simulink model "Mcity"  (R2019a)
settings: Solver=VariableStepAuto  StartTime=0.0  StopTime=100  RelTol=1e-3
undefined symbols (not defined in the file or in its folder): m, n
settings Model: Creator=nebneBgnahZ  LastModifiedBy=nebneBgnahZ
settings DataIOCC: ReturnWorkspaceOutputs=off
settings DebuggingCC: ArithmeticOperatorsInVariantConditions=warning
settings SFSimCC: SimUseLocalCustomCode=off
settings RTWCC: RTWUseLocalCustomCode=off
settings CodeAppCC: StateflowObjectComments=on

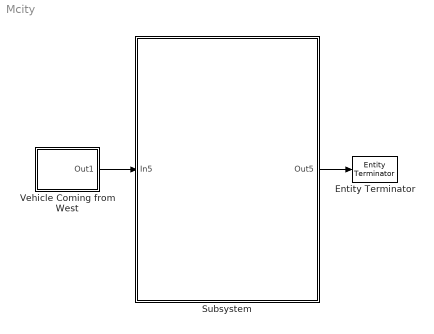
== system Mcity ==
  Entity Terminator : EntityTerminator  InputPortMessageModes=m
      mask Display: image('figs/CAV2.png');
  Subsystem : Subsystem
      mask Display: image('figs/Mcity Map - High Res.jpg');
  Vehicle Coming from West : Subsystem  mask(Connected Automated Vehicles (CAVs)){modelpopup=Basic model, umin=[], umax=[], vmin=[], vmax=[], length=0, cf=0, cr=0, lf=0, lr=0}
      mask prompts: modelpopup "Vehicle Model Selection"; umin "Maximum Deceleration"; umax "Maximum Acceleration"; vmin "Minimum Speed"; vmax "Maximum Speed"; cf "Front Tire Cornering Stiffness"; cr "Rear Tire Cornering Stiffness"; lf "Distance from CoG to Front Axels"; lr "Distance from CoG to Rear Axels"
      mask help: Vehicles, assumed to be CAVs, should possess the ability to communicate with the controller, the coordinator, and other vehicles in the network. CAVs can differ in driver models, for instance, motion dynamics, control mechanism, and fuel consumption dynamics.
      mask TypeOptions modelpopup: Basic model | Kinematic model | Dynamic model | User-defined
      mask Callback modelpopup:
      | % Get the mask parameter values. This is a cell
      | %   array of character vectors.
      | maskStr = get_param(gcb,'modelpopup');
      | 
      | % The pop-up menu is the first mask parameter.
      | %   Check the value selected in the pop-up
      | if strcmp(maskStr(1),'U')
      | 
      | 
      |     % Set the visibility of both parameters on when
      |     %   User-defined is selected in the pop-up.
      | 
      |     set_param(gcb,'MaskVisibilities',{'on';'on';'on';'on';'on';'on';'on';'on';'on';'on';}),
      | 
      | elseif strcmp(maskStr(1),'B')
      | 
      |     % Turn off the visibility of the Value field
      |     %   when User-defined is not selected.
      | 
      |     set_param(gcb,'MaskVisibilities',{'on';'on';'on';'on';'on';'off';'off';'off';'off';'off';}),
      | 
      |     % Set the character vector in the Values field equal to the
      |     % character vector selected in the Gain pop-up menu.
      | 
      |     %maskStr{2}=maskStr{1};
      | 
      | 
      | elseif strcmp(maskStr(1),'K')
      | 
      |     set_param(gcb,'MaskVisibilities',{'on';'on';'on';'on';'on';'on';'off';'off';'off';'off';}),
      | 
      | else
      | 
      |     set_param(gcb,'MaskVisibilities',{'on';'on';'on';'on';'on';'off';'on';'on';'on';'on';}),
      | 
      | end
      mask Display: image('figs/CAV.png');
  wires:
  Subsystem/1(Out5) -> Entity Terminator/1
  Vehicle Coming from West/1(Out1) -> Subsystem/1(In5)

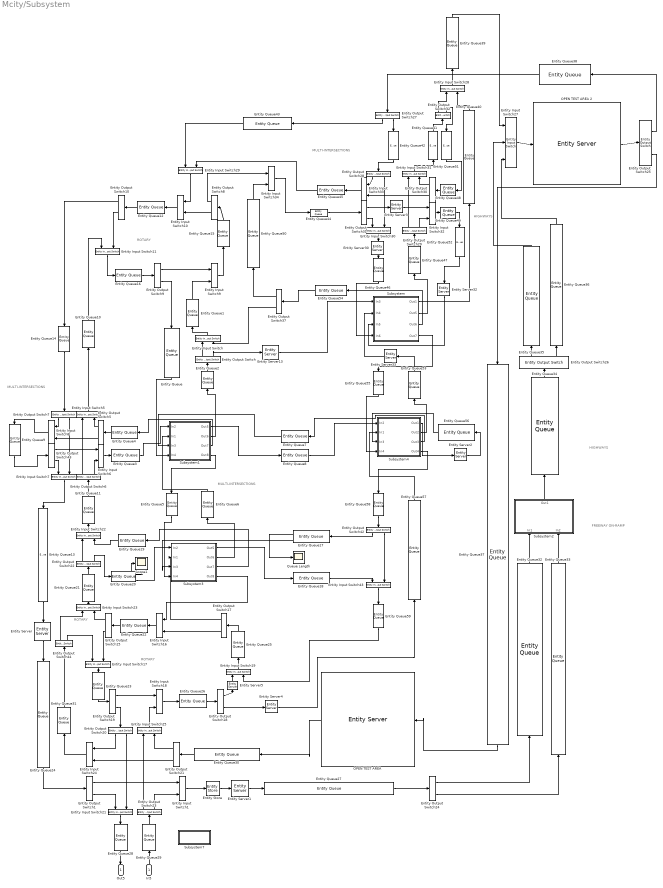
== system Mcity/Subsystem ==
  note: FREEWAY
      | ON-RAMP
  note: HIGHWAYS
  note: MULTI-INTERSECTIONS
  note: ROTARY
  note: ROTARY
  note: ROTARY
  note: MULTI-INTERSECTIONS
  note: MULTI-INTERSECTIONS
  note: HIGHWAYS
  In5 : Inport
  Entity Input Switch{,1,5..11,16..19,21..25,28..34,43} (26 alike) : EntityInputSwitch  InputPortMessageModes=m,m  OutputPortMessageModes=m
  Entity Input Switch27 : EntityInputSwitch  InputPortMessageModes=m,m,m  OutputPortMessageModes=m  NumberInputPorts=3
      settings: InputPortMap=u1,u2,u3
  Entity Output Switch{,1,5..10,15,18,20..22,24..32,37,42..44} (26 alike) : EntityOutputSwitch  InputPortMessageModes=m  OutputPortMessageModes=m,m  SwitchingCriterion=Round robin  SwitchAttributeName=Attribute1
  Entity Output Switch17 : EntityOutputSwitch  InputPortMessageModes=m  OutputPortMessageModes=m,m  SwitchAttributeName=Attribute1
  Entity Output Switch19 : EntityOutputSwitch  InputPortMessageModes=m  OutputPortMessageModes=m,m  SwitchAttributeName=Attribute1
  Entity Output Switch23 : EntityOutputSwitch  InputPortMessageModes=m  OutputPortMessageModes=m,m  SwitchingCriterion=Round robin  SwitchAttributeName=Lane
  Entity Queue{,1..16,19,21..26,28,30..31,35..59} (52 alike) : EntityQueue  InputPortMessageModes=m  OutputPortMessageModes=m
      settings: OutputPortMap=o5
  Entity Queue17 : EntityQueue  InputPortMessageModes=m  OutputPortMessageModes=n,m  Capacity=15  NumberEntitiesInBlock=on
      settings: OutputPortMap=o1,o5
  Entity Queue18 : EntityQueue  InputPortMessageModes=m  OutputPortMessageModes=m  Capacity=15
      settings: OutputPortMap=o5
  Entity Queue20 : EntityQueue  InputPortMessageModes=m  OutputPortMessageModes=n,m  AverageQueueLength=on
      settings: OutputPortMap=o3,o5
  Entity Queue{27,29,32..34} (5 alike) : EntityQueue  InputPortMessageModes=m  OutputPortMessageModes=m  Capacity=Inf
      settings: OutputPortMap=o5
  Entity Server{,3,5,13,30,32..33} (7 alike) : EntityServer  InputPortMessageModes=m  OutputPortMessageModes=m  Capacity=Inf  ServiceTimeValue=2.5
  Entity Server1 : EntityServer  InputPortMessageModes=m  OutputPortMessageModes=m  Capacity=1  ServiceTimeValue=2
  Entity Server2 : EntityServer  InputPortMessageModes=m  OutputPortMessageModes=m  Capacity=Inf  ServiceTimeValue=5
  Entity Server4 : EntityServer  InputPortMessageModes=m  OutputPortMessageModes=m  Capacity=Inf  ServiceTimeValue=5
  Entity Store : EntityStore  InputPortMessageModes=m  OutputPortMessageModes=m  Capacity=100
      settings: OutputPortMap=o4
  OPEN TEST AREA : EntityServer  InputPortMessageModes=m  OutputPortMessageModes=m  Capacity=200
  "OPEN TEST AREA 2 " : EntityServer  InputPortMessageModes=m  OutputPortMessageModes=m  Capacity=200
  Queue Length : Scope
  Scope1 : Scope
  Subsystem : Subsystem
      mask Display:
      | %image('figs/tlc.png');
      | 
      | fprintf('Signalized\n\n');
      | fprintf('\n\nIntersection 1');
  Subsystem1 : Subsystem
      mask Display:
      | %image('figs/unsignalized.png');
      | fprintf('Unsignalized\n\n');
      | fprintf('\n\nIntersection 1');
  Subsystem2 : Subsystem
      mask Display:
      | %image('figs/merge.png');
      | %image('figs/unsignalized.png');
      | fprintf('Freeway\n\n');
      | fprintf('\n\n On-Ramp');
  Subsystem3 : Subsystem
      mask Display:
      | %image('figs/tlc.png');
      | fprintf('Signalized\n\n');
      | fprintf('\n\nIntersection 2');
  Subsystem4 : Subsystem
      mask Display:
      | %image('figs/unsignalized.png');
      | fprintf('Unsignalized\n\n');
      | fprintf('\n\nIntersection 2');
  Subsystem7 : Subsystem
      settings: OpenFcn=init_func
      mask Display: disp('init');
  Out5 : Outport
  wires:
  Subsystem1/4(Out8) -> Entity Queue5/1
  Entity Input Switch10/1 -> Entity Queue12/1
  Entity Output Switch8/2 -> Entity Input Switch10/2
  Entity Output Switch24/1 -> Entity Queue32/1
  Entity Output Switch24/2 -> Entity Queue33/1
  Entity Queue34/1 -> Entity Output Switch26/1
  Entity Output Switch26/1 -> Entity Queue35/1
  Entity Output Switch26/2 -> Entity Queue36/1
  Entity Input Switch27/1 -> "OPEN TEST AREA 2 "/1
  "OPEN TEST AREA 2 "/1 -> Entity Output Switch25/1
  Entity Queue37/1 -> OPEN TEST AREA/1
  Entity Output Switch25/1 -> Entity Queue38/1
  Entity Queue36/1 -> Entity Input Switch27/3
  Entity Queue35/1 -> Entity Input Switch27/2
  Entity Queue39/1 -> Entity Input Switch27/1
  Entity Input Switch28/1 -> Entity Queue39/1
  Entity Queue40/1 -> Entity Input Switch28/2
  Entity Queue41/1 -> Entity Output Switch32/1
  Entity Queue38/1 -> Entity Output Switch27/1
  Entity Output Switch27/1 -> Entity Queue43/1
  Entity Output Switch27/2 -> Entity Queue42/1
  Entity Input Switch29/1 -> Entity Input Switch10/1
  Entity Queue43/1 -> Entity Input Switch29/1
  Entity Output Switch31/2 -> Entity Input Switch30/1
  Entity Output Switch31/1 -> Entity Server3/1
  Entity Input Switch33/1 -> Entity Queue45/1
  Entity Output Switch28/1 -> Entity Input Switch33/1
  Entity Output Switch30/1 -> Entity Input Switch31/2
  Entity Output Switch30/2 -> Entity Input Switch33/2
  Entity Output Switch29/1 -> Entity Input Switch31/1
  Entity Input Switch32/1 -> Entity Queue49/1
  Entity Queue48/1 -> Entity Output Switch30/1
  Entity Output Switch29/2 -> Entity Input Switch32/2
  Entity Queue45/1 -> Entity Input Switch29/2
  Entity Queue47/1 -> Entity Output Switch29/1
  Entity Queue42/1 -> Entity Output Switch28/1
  Entity Input Switch31/1 -> Entity Queue41/1
  Entity Queue50/1 -> Entity Input Switch34/2
  Entity Input Switch34/1 -> Entity Queue44/1
  Entity Output Switch32/1 -> Entity Input Switch28/1
  Entity Output Switch32/2 -> Entity Queue51/1
  Entity Queue51/1 -> Entity Queue48/1
  Entity Queue49/1 -> Entity Queue52/1
  Entity Queue54/1 -> Entity Output Switch37/1
  Entity Output Switch37/1 -> Entity Queue50/1
  Subsystem4/2(Out2) -> Entity Queue53/1
  Subsystem4/1(Out1) -> Entity Server2/1
  Subsystem4/4(Out4) -> Entity Queue58/1
  Entity Queue58/1 -> Entity Output Switch42/1
  Entity Input Switch43/1 -> Entity Queue59/1
  Entity Output Switch8/1 -> Entity Input Switch34/1
  Entity Output Switch10/2 -> Entity Input Switch11/2
  Entity Input Switch11/1 -> Entity Queue16/1
  Entity Queue16/1 -> Entity Output Switch9/1
  Entity Queue12/1 -> Entity Output Switch10/1
  Entity Queue15/1 -> Entity Output Switch8/1
  Entity Input Switch9/1 -> Entity Queue15/1
  Entity Input Switch16/1 -> Entity Queue22/1
  Entity Queue22/1 -> Entity Output Switch15/1
  Entity Input Switch17/1 -> Entity Queue23/1
  Entity Output Switch17/2 -> Entity Input Switch16/2
  Entity Queue26/1 -> Entity Output Switch18/1
  Entity Queue23/1 -> Entity Output Switch19/1
  Entity Input Switch19/1 -> Entity Queue25/1
  Entity Queue25/1 -> Entity Output Switch17/1
  Entity Queue30/1 -> Entity Output Switch21/1
  Entity Input Switch22/1 -> Entity Queue11/1
  Entity Output Switch22/1 -> Entity Input Switch22/1
  Entity Queue21/1 -> Entity Output Switch22/1
  Entity Input Switch23/1 -> Entity Queue21/1
  Entity Output Switch15/1 -> Entity Input Switch23/2
  Entity Queue31/1 -> Entity Output Switch44/1
  Entity Queue29/1 -> Entity Output Switch23/1
  Entity Input Switch21/1 -> Entity Queue28/1
  Entity Queue28/1 -> Out5/1
  In5/1 -> Entity Queue29/1
  Entity Output Switch5/2 -> Entity Input Switch8/2
  Entity Input Switch7/1 -> Entity Queue13/1
  Entity Output Switch7/2 -> Entity Input Switch7/2
  Entity Output Switch6/1 -> Entity Input Switch5/1
  Entity Output Switch9/1 -> Entity Input Switch9/1
  Entity Input Switch/1 -> Entity Queue1/1
  Subsystem1/2(Out6) -> Entity Queue2/1
  Entity Output Switch37/2 -> Entity Input Switch/2
  Entity Output Switch/2 -> Entity Server13/1
  Subsystem1/3(Out7) -> Entity Queue4/1
  Entity Queue2/1 -> Entity Output Switch/1
  Entity Output Switch9/2 -> Entity Queue/1
  Entity Queue1/1 -> Entity Input Switch9/2
  Entity Queue7/1 -> Subsystem1/3(In3)
  Entity Output Switch/1 -> Entity Input Switch/1
  Entity Queue4/1 -> Entity Output Switch5/1
  Entity Input Switch5/1 -> Entity Queue10/1
  Entity Output Switch5/1 -> Entity Input Switch5/2
  Entity Input Switch6/1 -> Entity Queue3/1
  Entity Output Switch6/2 -> Entity Input Switch6/2
  Entity Queue11/1 -> Entity Output Switch6/1
  Entity Queue9/1 -> Entity Output Switch43/1
  Entity Output Switch7/1 -> Entity Input Switch8/1
  Entity Queue14/1 -> Entity Output Switch7/1
  Entity Output Switch43/1 -> Entity Input Switch6/1
  Entity Output Switch43/2 -> Entity Input Switch7/1
  Entity Output Switch44/1 -> Entity Input Switch23/1
  Subsystem2/1(Out1) -> Entity Queue34/1
  Entity Queue32/1 -> Subsystem2/1(In1)
  Entity Queue33/1 -> Subsystem2/2(In2)
  Entity Queue13/1 -> Entity Server/1
  Entity Server/1 -> Entity Queue24/1
  OPEN TEST AREA/1 -> Entity Queue30/1
  Entity Output Switch10/1 -> Entity Queue14/1
  Entity Queue10/1 -> Entity Input Switch11/1
  Subsystem/1(Out1) -> Entity Queue40/1
  Entity Input Switch8/1 -> Entity Queue9/1
  Entity Output Switch15/2 -> Entity Input Switch17/2
  Entity Output Switch44/2 -> Entity Input Switch17/1
  Entity Input Switch24/1 -> Entity Queue31/1
  Entity Output Switch19/1 -> Entity Input Switch18/1
  Entity Input Switch18/1 -> Entity Queue26/1
  Entity Output Switch19/2 -> Entity Output Switch20/1
  Entity Input Switch25/1 -> Entity Input Switch18/2
  Entity Output Switch20/1 -> Entity Input Switch24/1
  Entity Output Switch21/1 -> Entity Input Switch25/2
  Entity Output Switch20/2 -> Entity Input Switch21/2
  Entity Output Switch23/1 -> Entity Input Switch25/1
  Subsystem/2(Out5) -> Entity Queue47/1
  Subsystem/3(Out6) -> Entity Queue54/1
  Subsystem/4(Out7) -> Entity Queue55/1
  Entity Server13/1 -> Subsystem/1(In3)
  Entity Queue53/1 -> Entity Server33/1
  Entity Queue52/1 -> Entity Server32/1
  Entity Queue46/1 -> Subsystem/4(In6)
  Entity Output Switch28/2 -> Entity Input Switch30/2
  Entity Queue44/1 -> Entity Output Switch31/1
  Entity Server32/1 -> Subsystem/3(In5)
  Entity Server33/1 -> Subsystem/2(In4)
  Entity Input Switch30/1 -> Entity Server30/1
  Entity Server30/1 -> Entity Queue46/1
  Entity Output Switch21/2 -> Entity Input Switch24/2
  Entity Queue59/1 -> Entity Input Switch19/2
  Entity Output Switch18/2 -> Entity Server4/1
  Subsystem4/3(Out3) -> Entity Queue7/1
  Entity Output Switch25/2 -> Entity Queue37/1
  Entity Server2/1 -> Entity Queue56/1
  Entity Server3/1 -> Entity Input Switch32/1
  Entity Server4/1 -> Entity Queue57/1
  Entity Server5/1 -> Entity Input Switch19/1
  Entity Output Switch18/1 -> Entity Server5/1
  Entity Queue20/1 -> Scope1/1
  Entity Queue17/1 -> Queue Length/1
  Entity Queue5/1 -> Subsystem3/4(In4)
  Subsystem3/4(Out8) -> Entity Input Switch16/1
  Entity Queue17/2 -> Subsystem3/3(In3)
  Subsystem3/3(Out7) -> Entity Queue19/1
  Entity Output Switch42/1 -> Entity Queue17/1
  Entity Queue20/2 -> Subsystem3/1(In2)
  Subsystem3/2(Out6) -> Entity Queue6/1
  Entity Queue19/1 -> Entity Input Switch22/2
  Entity Output Switch22/2 -> Entity Queue20/1
  Entity Output Switch17/1 -> Subsystem3/2(In1)
  Entity Queue18/1 -> Entity Input Switch43/1
  Subsystem3/1(Out5) -> Entity Queue18/1
  Entity Output Switch42/2 -> Entity Input Switch43/2
  Entity Queue3/1 -> Subsystem1/1(In2)
  Entity Queue6/1 -> Subsystem1/2(In1)
  Entity Queue/1 -> Subsystem1/4(In4)
  Subsystem1/1(Out5) -> Entity Queue8/1
  Entity Queue8/1 -> Subsystem4/1(In2)
  Entity Queue57/1 -> Subsystem4/2(In1)
  Entity Queue56/1 -> Subsystem4/3(In3)
  Entity Queue55/1 -> Subsystem4/4(In4)
  Entity Queue24/1 -> Entity Output Switch1/1
  Entity Output Switch1/2 -> Entity Input Switch21/1
  Entity Input Switch1/1 -> Entity Store/1
  Entity Output Switch1/1 -> Entity Input Switch1/1
  Entity Output Switch23/2 -> Entity Input Switch1/2
  Entity Queue27/1 -> Entity Output Switch24/1
  Entity Server1/1 -> Entity Queue27/1
  Entity Store/1 -> Entity Server1/1

== system Mcity/Vehicle Coming from West ==
  "CAV generator " : EntityGenerator  DialogController=slde.AttributeBlockDialog  OutputPortMessageModes=m  TimeSource=MATLAB action  IntergenerationTimeAction=|  GenerateAction=entity.Speed = 9 + 2 * rand();  AttributeName=ID|Speed|ArrivalTime|FinalSpeed|FinalTime|Position|Lane|Destination|Acceleration|coe  AttributeInitialValue=0|1|1|1|1|0|1|1|1|[0 0 0 0]  EntityType=Bus object  EntityTypeName=CAV
      | mean = 1.5;
      | dt = 1.5 - mean*log(rand());
  Out1 : Outport
  wires:
  "CAV generator "/1 -> Out1/1

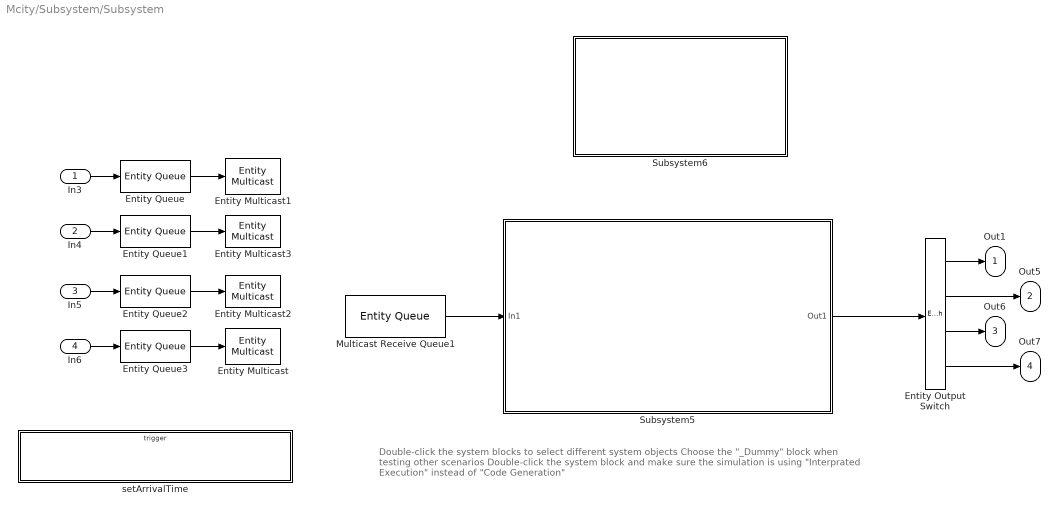
== system Mcity/Subsystem/Subsystem ==
  note: Double-click the system blocks to select different system objects
      | Choose the "_Dummy" block when testing other scenarios
      | Double-click the system block and make sure the simulation is using "Interprated Execution" instead of "Code Generation"
  In3 : Inport
  In4 : Inport  Port=2
  In5 : Inport  Port=3
  In6 : Inport  Port=4
  Entity Output Switch : EntityOutputSwitch  InputPortMessageModes=m  OutputPortMessageModes=m,m,m,m  NumberOutputPorts=4  SwitchingCriterion=From attribute  SwitchAttributeName=Lane
      settings: OutputPortMap=o0,o1,o2,o3
  Entity Multicast{,1..3} (4 alike) : EntityMulticast  InputPortMessageModes=m  MulticastTag=sig_1_CAV
  Entity Queue : EntityQueue  InputPortMessageModes=m  OutputPortMessageModes=m  Capacity=Inf  EntryAction=|
      | [entity.ArrivalTime,...
      |     entity.ID] = sig_int_setArrivalTime();
      | entity.Lane = 1;
      | entity.Speed = 8 + 4 * rand();
      | entity.Position = 0;
      settings: OutputPortMap=o5
  Entity Queue1 : EntityQueue  InputPortMessageModes=m  OutputPortMessageModes=m  Capacity=Inf  EntryAction=|
      | [entity.ArrivalTime,...
      |     entity.ID] = sig_int_setArrivalTime();
      | entity.Lane = 2;
      | entity.Speed = 9 + 3 * rand();
      | entity.Position = 0;
      settings: OutputPortMap=o5
  Entity Queue2 : EntityQueue  InputPortMessageModes=m  OutputPortMessageModes=m  Capacity=Inf  EntryAction=|
      | [entity.ArrivalTime,...
      |     entity.ID] = sig_int_setArrivalTime();
      | entity.Lane = 3;
      | entity.Speed = 8 + 4 * rand();
      | entity.Position = 0;
      settings: OutputPortMap=o5
  Entity Queue3 : EntityQueue  InputPortMessageModes=m  OutputPortMessageModes=m  Capacity=Inf  EntryAction=|
      | [entity.ArrivalTime,...
      |     entity.ID] = sig_int_setArrivalTime();
      | entity.Lane = 4;
      | entity.Speed = 9 + 3 * rand();
      | entity.Position = 0;
      settings: OutputPortMap=o5
  Multicast Receive Queue1 : EntityQueue  OutputPortMessageModes=m  Capacity=200  EntityArrivalSource=Multicast  MulticastTag=sig_1_CAV  EntryAction=|
      | rann = rand();
      | if rann < 0.5
      |     entity.Type = 0;
      | else
      |     entity.Type = 1;
      | end
      settings: OutputPortMap=o5
  Subsystem5 : Subsystem
      mask Display:
      | %image('figs/controller.jpg');
      | disp('Control Zone')
  Subsystem6 : Subsystem
      mask Display: disp('Traffic Signal')
  setArrivalTime : Subsystem  TreatAsAtomicUnit=on
  Out1 : Outport
  Out5 : Outport  Port=2
  Out6 : Outport  Port=3
  Out7 : Outport  Port=4
  wires:
  Subsystem5/1(Out1) -> Entity Output Switch/1
  In3/1 -> Entity Queue/1
  In4/1 -> Entity Queue1/1
  In6/1 -> Entity Queue3/1
  In5/1 -> Entity Queue2/1
  Entity Output Switch/1 -> Out1/1
  Entity Output Switch/2 -> Out5/1
  Entity Output Switch/3 -> Out6/1
  Entity Output Switch/4 -> Out7/1
  Entity Queue/1 -> Entity Multicast1/1
  Entity Queue1/1 -> Entity Multicast3/1
  Entity Queue2/1 -> Entity Multicast2/1
  Entity Queue3/1 -> Entity Multicast/1
  Multicast Receive Queue1/1 -> Subsystem5/1(In1)

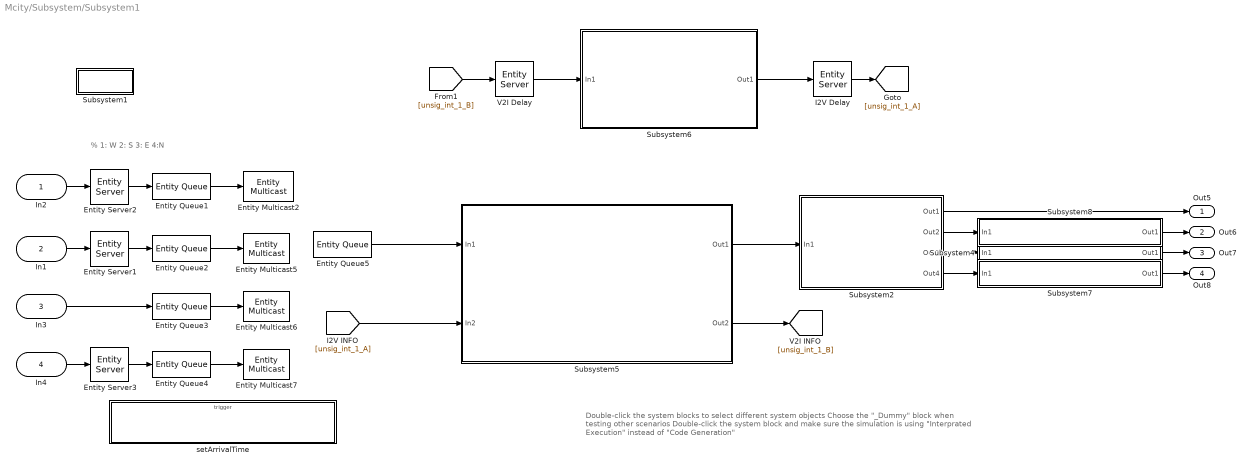
== system Mcity/Subsystem/Subsystem1 ==
  note: % 1: W 2: S 3: E 4:N
  note: Double-click the system blocks to select different system objects
      | Choose the "_Dummy" block when testing other scenarios
      | Double-click the system block and make sure the simulation is using "Interprated Execution" instead of "Code Generation"
  In2 : Inport
  In1 : Inport  Port=2
  In3 : Inport  Port=3
  In4 : Inport  Port=4
  Entity Multicast{2,5..7} (4 alike) : EntityMulticast  InputPortMessageModes=m  MulticastTag=unsig_1_CAV
  Entity Queue1 : EntityQueue  InputPortMessageModes=m  OutputPortMessageModes=m  Capacity=Inf  EntryAction=|
      | entity.Lane = 1;
      | [entity.ArrivalTime,...
      |     entity.ID] = unsig_int_1_setArrivalTime();
      | entity.FinalSpeed = 10;
      | entity.Position = 0;
      | entity.Intersection = 1;
      settings: OutputPortMap=o5
  Entity Queue2 : EntityQueue  InputPortMessageModes=m  OutputPortMessageModes=m  Capacity=Inf  EntryAction=|
      | entity.Lane = 2;
      | [entity.ArrivalTime,...
      |     entity.ID] = unsig_int_1_setArrivalTime();
      | entity.FinalSpeed = 10;
      | entity.Position = 0;
      | entity.Intersection = 1;
      settings: OutputPortMap=o5
  Entity Queue3 : EntityQueue  InputPortMessageModes=m  OutputPortMessageModes=m  Capacity=Inf  EntryAction=|
      | entity.Lane = 3;
      | [entity.ArrivalTime,...
      |     entity.ID] = unsig_int_1_setArrivalTime();
      | entity.FinalSpeed = 10;
      | entity.Position = 0;
      | entity.Intersection = 1;
      settings: OutputPortMap=o5
  Entity Queue4 : EntityQueue  InputPortMessageModes=m  OutputPortMessageModes=m  Capacity=Inf  EntryAction=|
      | entity.Lane = 4;
      | [entity.ArrivalTime,...
      |     entity.ID] = unsig_int_1_setArrivalTime();
      | entity.FinalSpeed = 10;
      | entity.Position = 0;
      | entity.Intersection = 1;
      settings: OutputPortMap=o5
  Entity Queue5 : EntityQueue  OutputPortMessageModes=m  Capacity=400  EntityArrivalSource=Multicast  MulticastTag=unsig_1_CAV  EntryAction=entity.Intersection = 1;
      settings: OutputPortMap=o5
  Entity Server1 : EntityServer  InputPortMessageModes=m  OutputPortMessageModes=m  Capacity=Inf  ServiceTimeValue=2.5
  Entity Server2 : EntityServer  InputPortMessageModes=m  OutputPortMessageModes=m  Capacity=Inf  ServiceTimeValue=2.5
  Entity Server3 : EntityServer  InputPortMessageModes=m  OutputPortMessageModes=m  Capacity=Inf  ServiceTimeValue=2.5
  I2V Delay : EntityServer  InputPortMessageModes=m  OutputPortMessageModes=m  Capacity=Inf  ServiceTimeValue=0.01
  Subsystem1 : Subsystem
      settings: OpenFcn=init_func
      mask Display: disp('init');
  Subsystem2 : Subsystem
      mask Display: disp('Merging Zone')
  Subsystem4 : Subsystem
      mask Display: disp('Leaving the network')
  Subsystem5 : Subsystem
      mask Display:
      | %image('figs/controller.jpg');
      | disp('Control Zone')
  Subsystem6 : Subsystem
      mask Display:
      | %image('figs/coordinator.jpg');
      | disp('Coordinator')
  Subsystem7 : Subsystem
      mask Display: disp('Leaving the network')
  Subsystem8 : Subsystem
      mask Display: disp('Leaving the network')
  V2I Delay : EntityServer  InputPortMessageModes=m  OutputPortMessageModes=m  Capacity=Inf  ServiceTimeValue=0.01
  setArrivalTime : Subsystem  TreatAsAtomicUnit=on
  Out5 : Outport
  Out6 : Outport  Port=2
  Out7 : Outport  Port=3
  Out8 : Outport  Port=4
  wires:
  [unsig_int_1_B] -> V2I Delay/1
  Entity Queue4/1 -> Entity Multicast7/1
  Subsystem2/2(Out2) -> Subsystem8/1(In1)
  Entity Queue3/1 -> Entity Multicast6/1
  Subsystem5/1(Out1) -> Subsystem2/1(In1)
  Entity Queue1/1 -> Entity Multicast2/1
  Subsystem2/3(Out3) -> Subsystem4/1(In1)
  In4/1 -> Entity Server3/1
  In1/1 -> Entity Server1/1
  Subsystem4/1(Out1) -> Out7/1
  Entity Queue2/1 -> Entity Multicast5/1
  Subsystem2/1(Out1) -> Out5/1
  V2I Delay/1 -> Subsystem6/1(In1)
  Subsystem2/4(Out4) -> Subsystem7/1(In1)
  Subsystem7/1(Out1) -> Out8/1
  Subsystem5/2(Out2) -> [unsig_int_1_B]
  Subsystem8/1(Out1) -> Out6/1
  Subsystem6/1(Out1) -> I2V Delay/1
  I2V Delay/1 -> [unsig_int_1_A]
  Entity Queue5/1 -> Subsystem5/1(In1)
  [unsig_int_1_A] -> Subsystem5/2(In2)
  Entity Server1/1 -> Entity Queue2/1
  Entity Server3/1 -> Entity Queue4/1
  In2/1 -> Entity Server2/1
  Entity Server2/1 -> Entity Queue1/1
  In3/1 -> Entity Queue3/1

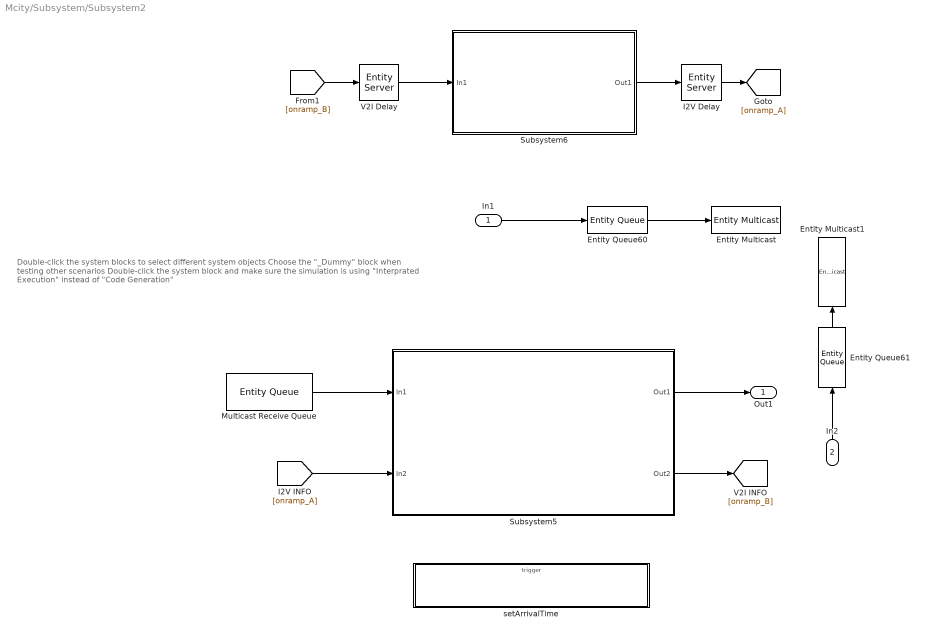
== system Mcity/Subsystem/Subsystem2 ==
  note: Double-click the system blocks to select different system objects
      | Choose the "_Dummy" block when testing other scenarios
      | Double-click the system block and make sure the simulation is using "Interprated Execution" instead of "Code Generation"
  In1 : Inport
  In2 : Inport  Port=2
  Entity Multicast : EntityMulticast  InputPortMessageModes=m  MulticastTag=onramp_CAV
  Entity Multicast1 : EntityMulticast  InputPortMessageModes=m  MulticastTag=onramp_CAV
  Entity Queue60 : EntityQueue  InputPortMessageModes=m  OutputPortMessageModes=m  Capacity=20  EntryAction=|
      | [entity.ArrivalTime,...
      |     entity.ID] = onramp_setArrivalTime();
      | entity.Lane = 1;
      | entity.Speed = 8 + 4 * rand();
      | entity.Position = 0;
      | entity.FinalSpeed = 10;
      settings: OutputPortMap=o5
  Entity Queue61 : EntityQueue  InputPortMessageModes=m  OutputPortMessageModes=m  Capacity=20  EntryAction=|
      | [entity.ArrivalTime,...
      |     entity.ID] = onramp_setArrivalTime();
      | entity.Lane = 2;
      | entity.Speed = 8 + 4 * rand();
      | entity.Position = 0;
      | entity.FinalSpeed = 10;
      settings: OutputPortMap=o5
  I2V Delay : EntityServer  InputPortMessageModes=m  OutputPortMessageModes=m  Capacity=Inf  ServiceTimeValue=0.01
  Multicast Receive Queue : EntityQueue  OutputPortMessageModes=m  Capacity=100  EntityArrivalSource=Multicast  MulticastTag=onramp_CAV
      settings: OutputPortMap=o5
  Subsystem5 : Subsystem
      mask Display:
      | %image('figs/controller.jpg');
      | disp('MERGING')
  Subsystem6 : Subsystem
      mask Display:
      | %image('figs/coordinator.jpg');
      | disp('Coordinator')
  V2I Delay : EntityServer  InputPortMessageModes=m  OutputPortMessageModes=m  Capacity=Inf  ServiceTimeValue=0.01
  setArrivalTime : Subsystem  TreatAsAtomicUnit=on
  Out1 : Outport
  wires:
  [onramp_B] -> V2I Delay/1
  Subsystem5/2(Out2) -> [onramp_B]
  In1/1 -> Entity Queue60/1
  Subsystem6/1(Out1) -> I2V Delay/1
  [onramp_A] -> Subsystem5/2(In2)
  Subsystem5/1(Out1) -> Out1/1
  In2/1 -> Entity Queue61/1
  I2V Delay/1 -> [onramp_A]
  V2I Delay/1 -> Subsystem6/1(In1)
  Entity Queue60/1 -> Entity Multicast/1
  Entity Queue61/1 -> Entity Multicast1/1
  Multicast Receive Queue/1 -> Subsystem5/1(In1)

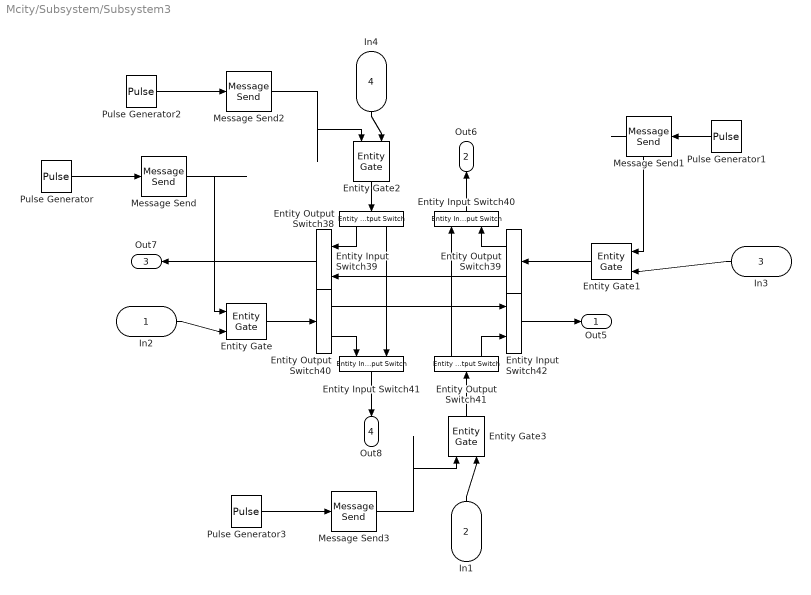
== system Mcity/Subsystem/Subsystem3 ==
  In2 : Inport
  In1 : Inport  Port=2
  In3 : Inport  Port=3
  In4 : Inport  Port=4
  Entity Input Switch{39..42} (4 alike) : EntityInputSwitch  InputPortMessageModes=m,m  OutputPortMessageModes=m
  Entity Output Switch{38..41} (4 alike) : EntityOutputSwitch  InputPortMessageModes=m  OutputPortMessageModes=m,m  SwitchingCriterion=Round robin  SwitchAttributeName=Attribute1
  Entity Gate{,1..3} (4 alike) : EntityGate  InputPortMessageModes=m,m  OutputPortMessageModes=m
  Message Send{,1..3} (4 alike) : MessageSend  OutputPortMessageModes=m
      settings: InputPortMap=u1
  Pulse Generator : DiscretePulseGenerator  PulseType=Time based  Period=30  PulseWidth=50
  Pulse Generator1 : DiscretePulseGenerator  PulseType=Time based  Period=30  PulseWidth=50
  Pulse Generator2 : DiscretePulseGenerator  PulseType=Time based  Period=30  PulseWidth=50  PhaseDelay=15  VectorParams1D=off
  Pulse Generator3 : DiscretePulseGenerator  PulseType=Time based  Period=30  PulseWidth=50  PhaseDelay=15  VectorParams1D=off
  Out5 : Outport
  Out6 : Outport  Port=2
  Out7 : Outport  Port=3
  Out8 : Outport  Port=4
  wires:
  Entity Input Switch40/1 -> Out6/1
  Entity Output Switch41/1 -> Entity Input Switch40/1
  Entity Output Switch40/2 -> Entity Input Switch41/1
  Entity Output Switch40/1 -> Entity Input Switch42/1
  In3/1 -> Entity Gate1/2
  Entity Output Switch39/2 -> Entity Input Switch39/2
  Entity Output Switch38/2 -> Entity Input Switch41/2
  Entity Output Switch41/2 -> Entity Input Switch42/2
  Entity Output Switch39/1 -> Entity Input Switch40/2
  Entity Output Switch38/1 -> Entity Input Switch39/1
  Entity Input Switch42/1 -> Out5/1
  Entity Input Switch39/1 -> Out7/1
  Entity Input Switch41/1 -> Out8/1
  Entity Gate/1 -> Entity Output Switch40/1
  Pulse Generator/1 -> Message Send/1
  Message Send/1 -> Entity Gate/1
  In2/1 -> Entity Gate/2
  Entity Gate1/1 -> Entity Output Switch39/1
  Message Send1/1 -> Entity Gate1/1
  Pulse Generator1/1 -> Message Send1/1
  In4/1 -> Entity Gate2/2
  Entity Gate2/1 -> Entity Output Switch38/1
  Pulse Generator2/1 -> Message Send2/1
  Message Send2/1 -> Entity Gate2/1
  Pulse Generator3/1 -> Message Send3/1
  In1/1 -> Entity Gate3/2
  Message Send3/1 -> Entity Gate3/1
  Entity Gate3/1 -> Entity Output Switch41/1

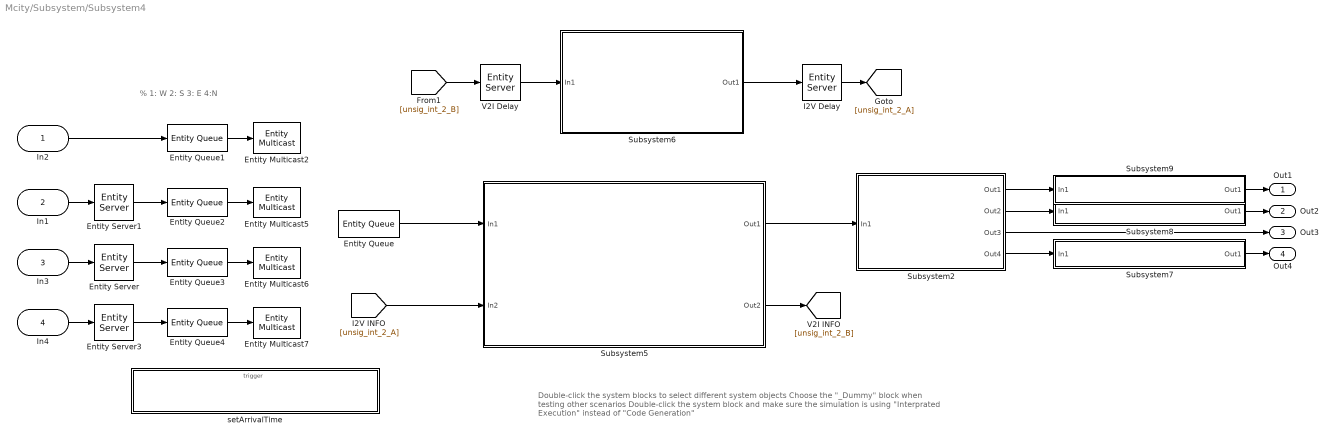
== system Mcity/Subsystem/Subsystem4 ==
  note: % 1: W 2: S 3: E 4:N
  note: Double-click the system blocks to select different system objects
      | Choose the "_Dummy" block when testing other scenarios
      | Double-click the system block and make sure the simulation is using "Interprated Execution" instead of "Code Generation"
  In2 : Inport
  In1 : Inport  Port=2
  In3 : Inport  Port=3
  In4 : Inport  Port=4
  Entity Multicast{2,5..7} (4 alike) : EntityMulticast  InputPortMessageModes=m  MulticastTag=unsig_int_2_CAV
  Entity Queue : EntityQueue  OutputPortMessageModes=m  Capacity=400  EntityArrivalSource=Multicast  MulticastTag=unsig_int_2_CAV
      settings: OutputPortMap=o5
  Entity Queue1 : EntityQueue  InputPortMessageModes=m  OutputPortMessageModes=m  Capacity=Inf  EntryAction=|
      | entity.Lane = 1;
      | [entity.ArrivalTime,...
      |     entity.ID] = unsig_int_2_setArrivalTime();
      | entity.FinalSpeed = 10;
      | entity.Position = 0;
      | entity.Intersection = 2;
      settings: OutputPortMap=o5
  Entity Queue2 : EntityQueue  InputPortMessageModes=m  OutputPortMessageModes=m  Capacity=Inf  EntryAction=|
      | entity.Lane = 2;
      | [entity.ArrivalTime,...
      |     entity.ID] = unsig_int_2_setArrivalTime();
      | entity.FinalSpeed = 10;
      | entity.Position = 0;
      | entity.Intersection = 2;
      settings: OutputPortMap=o5
  Entity Queue3 : EntityQueue  InputPortMessageModes=m  OutputPortMessageModes=m  Capacity=Inf  EntryAction=|
      | entity.Lane = 3;
      | [entity.ArrivalTime,...
      |     entity.ID] = unsig_int_2_setArrivalTime();
      | entity.FinalSpeed = 10;
      | entity.Position = 0;
      | entity.Intersection = 2;
      settings: OutputPortMap=o5
  Entity Queue4 : EntityQueue  InputPortMessageModes=m  OutputPortMessageModes=m  Capacity=Inf  EntryAction=|
      | entity.Lane = 4;
      | [entity.ArrivalTime,...
      |     entity.ID] = unsig_int_2_setArrivalTime();
      | entity.FinalSpeed = 10;
      | entity.Position = 0;
      | entity.Intersection = 2;
      settings: OutputPortMap=o5
  Entity Server : EntityServer  InputPortMessageModes=m  OutputPortMessageModes=m  Capacity=Inf  ServiceTimeValue=2.5
  Entity Server1 : EntityServer  InputPortMessageModes=m  OutputPortMessageModes=m  Capacity=Inf  ServiceTimeValue=2.5
  Entity Server3 : EntityServer  InputPortMessageModes=m  OutputPortMessageModes=m  Capacity=Inf  ServiceTimeValue=2.5
  I2V Delay : EntityServer  InputPortMessageModes=m  OutputPortMessageModes=m  Capacity=Inf  ServiceTimeValue=0.01
  Subsystem2 : Subsystem
      mask Display: disp('Merging Zone')
  Subsystem5 : Subsystem
      mask Display:
      | %image('figs/controller.jpg');
      | disp('Control Zone')
  Subsystem6 : Subsystem
      mask Display:
      | %image('figs/coordinator.jpg');
      | disp('Coordinator')
  Subsystem7 : Subsystem
      mask Display: disp('Leaving the network')
  Subsystem8 : Subsystem
      mask Display: disp('Leaving the network')
  Subsystem9 : Subsystem
      mask Display: disp('Leaving the network')
  V2I Delay : EntityServer  InputPortMessageModes=m  OutputPortMessageModes=m  Capacity=Inf  ServiceTimeValue=0.01
  setArrivalTime : Subsystem  TreatAsAtomicUnit=on
  Out1 : Outport
  Out2 : Outport  Port=2
  Out3 : Outport  Port=3
  Out4 : Outport  Port=4
  wires:
  [unsig_int_2_B] -> V2I Delay/1
  Entity Queue3/1 -> Entity Multicast6/1
  Entity Queue4/1 -> Entity Multicast7/1
  In4/1 -> Entity Server3/1
  Subsystem2/1(Out1) -> Subsystem9/1(In1)
  Subsystem7/1(Out1) -> Out4/1
  Subsystem5/2(Out2) -> [unsig_int_2_B]
  Subsystem9/1(Out1) -> Out1/1
  Entity Queue1/1 -> Entity Multicast2/1
  Entity Queue2/1 -> Entity Multicast5/1
  In1/1 -> Entity Server1/1
  Subsystem8/1(Out1) -> Out2/1
  Subsystem6/1(Out1) -> I2V Delay/1
  Subsystem2/3(Out3) -> Out3/1
  Subsystem5/1(Out1) -> Subsystem2/1(In1)
  [unsig_int_2_A] -> Subsystem5/2(In2)
  V2I Delay/1 -> Subsystem6/1(In1)
  Subsystem2/2(Out2) -> Subsystem8/1(In1)
  Subsystem2/4(Out4) -> Subsystem7/1(In1)
  Entity Queue/1 -> Subsystem5/1(In1)
  I2V Delay/1 -> [unsig_int_2_A]
  Entity Server1/1 -> Entity Queue2/1
  Entity Server3/1 -> Entity Queue4/1
  In3/1 -> Entity Server/1
  Entity Server/1 -> Entity Queue3/1
  In2/1 -> Entity Queue1/1

== system Mcity/Subsystem/Subsystem7 ==

== system Mcity/Subsystem/Subsystem/Subsystem5 ==
  note: Right-click the system block and select "Block Parameters (MATLAB Discrete Event Systems)"
      | Choose one of the controllers from
      | sig_int_Controller_OC (optimal control)
      | sig_int_Controller_IDM (intelligent driver model for human drivers)
      | sig_int_Controller_Mixed (optimal control for CAVs, intelligent driver model for non-CAVs)
      | sig_int_Controller_Dummy (choose this when testing other scenarios)
      | Double-click the system block and make sure the simulation is using "Interprated Execution" instead of "Code Generation"
  In1 : Inport
  MATLAB Discrete-Event System1 : MATLABDiscreteEventSystem  Description=Coordinator  InputPortMessageModes=m  OutputPortMessageModes=m  System=sig_int_Controller_Dummy  capacity=400  simulation_step=0.01  S=30  L=400  delta=10  SimulateUsing=Interpreted execution
      mask Type: sig_int_Controller_Dummy
      mask Display:
      | disp('CONTROL ZONE DUMMY');
      | port_label('input',1,'IN');
      | port_label('output',1,'OUT');
  Out1 : Outport
  wires:
  MATLAB Discrete-Event System1/1 -> Out1/1
  In1/1 -> MATLAB Discrete-Event System1/1

== system Mcity/Subsystem/Subsystem/Subsystem6 ==
  note: Right-click the system block and select "Block Parameters (MATLAB Discrete Event Systems)"
      | Choose one of the traffic signals from
      | sig_int_TrafficSignal
      | sig_int_TrafficSignal_Dummy (choose this when testing other scenarios)
      | Double-click the system block and make sure the simulation is using "Interprated Execution" instead of "Code Generation"
  " " : MATLABDiscreteEventSystem  System=sig_int_TrafficSignal_Dummy  capacity=100  SimulateUsing=Interpreted execution
      mask Type: sig_int_TrafficSignal_Dummy
      mask Display: disp('TRAFFIC SIGNAL DUMMY');

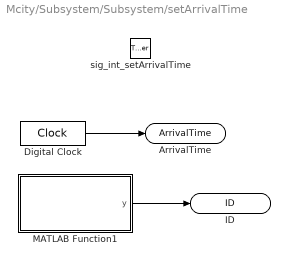
== system Mcity/Subsystem/Subsystem/setArrivalTime ==
  sig_int_setArrivalTime : TriggerPort  TriggerType=function-call  IsSimulinkFunction=on  FunctionName=sig_int_setArrivalTime  FunctionVisibility=scoped  VariantControl=Variant
  Digital Clock : DigitalClock  SampleTime=-1
  MATLAB Function1 : MATLAB Function  TreatAsAtomicUnit=on
  ArrivalTime : ArgOut  DisableCoverage=on  ArgumentName=ArrivalTime
  ID : ArgOut  DisableCoverage=on  Port=2  ArgumentName=ID
  wires:
  MATLAB Function1/1(y) -> ID/1
  Digital Clock/1 -> ArrivalTime/1

== system Mcity/Subsystem/Subsystem1/Subsystem1 ==

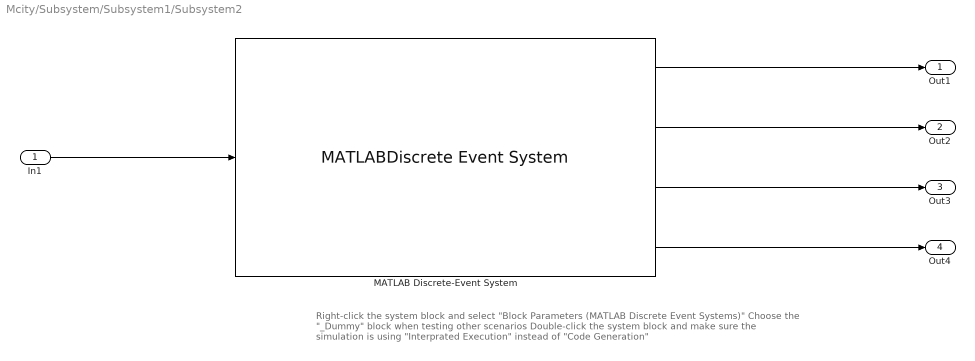
== system Mcity/Subsystem/Subsystem1/Subsystem2 ==
  note: Right-click the system block and select "Block Parameters (MATLAB Discrete Event Systems)"
      | Choose the "_Dummy" block when testing other scenarios
      | Double-click the system block and make sure the simulation is using "Interprated Execution" instead of "Code Generation"
  In1 : Inport
  MATLAB Discrete-Event System : MATLABDiscreteEventSystem  InputPortMessageModes=m  OutputPortMessageModes=m,m,m,m  System=unsig_int_1_MergingZoneCruiser_Dummy  capacity=200  SimulateUsing=Interpreted execution
      mask Type: unsig_int_1_MergingZoneCruiser_Dummy
      mask Display:
      | disp('THE MERGING ZONE');
      | port_label('input',1,'CAV');
      | port_label('output',1,'TO WEST');
      | port_label('output',2,'TO SOUTH');
      | port_label('output',3,'TO EAST');
      | port_label('output',4,'TO NORTH');
  Out1 : Outport
  Out2 : Outport  Port=2
  Out3 : Outport  Port=3
  Out4 : Outport  Port=4
  wires:
  MATLAB Discrete-Event System/1 -> Out1/1
  MATLAB Discrete-Event System/2 -> Out2/1
  MATLAB Discrete-Event System/3 -> Out3/1
  MATLAB Discrete-Event System/4 -> Out4/1
  In1/1 -> MATLAB Discrete-Event System/1

== system Mcity/Subsystem/Subsystem1/Subsystem4 ==
  In1 : Inport
  MATLAB Discrete-Event System : MATLABDiscreteEventSystem  InputPortMessageModes=m  OutputPortMessageModes=m  System=unsig_int_12_RoadSegment_Dummy  capacity=400  SimulateUsing=Interpreted execution
      mask Type: unsig_int_12_RoadSegment_Dummy
      mask Display:
      | disp('LEAVE THE INTERSECTION DUMMY');
      | port_label('input',1,'IN');
      | port_label('output',1,'OUT');
  Out1 : Outport
  wires:
  MATLAB Discrete-Event System/1 -> Out1/1
  In1/1 -> MATLAB Discrete-Event System/1

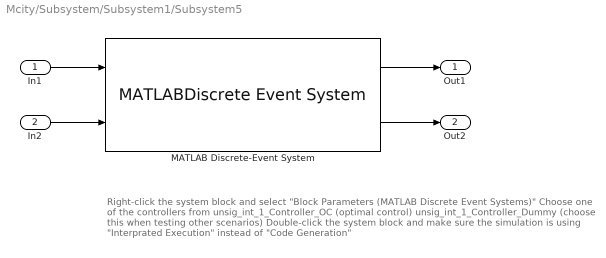
== system Mcity/Subsystem/Subsystem1/Subsystem5 ==
  note: Right-click the system block and select "Block Parameters (MATLAB Discrete Event Systems)"
      | Choose one of the controllers from
      | unsig_int_1_Controller_OC (optimal control)
      | unsig_int_1_Controller_Dummy (choose this when testing other scenarios)
      | Double-click the system block and make sure the simulation is using "Interprated Execution" instead of "Code Generation"
  In1 : Inport
  In2 : Inport  Port=2
  MATLAB Discrete-Event System : MATLABDiscreteEventSystem  InputPortMessageModes=m,m  OutputPortMessageModes=m,m  System=unsig_int_1_Controller_Dummy  capacity=400  SimulateUsing=Interpreted execution
      mask Type: unsig_int_1_Controller_Dummy
      mask Display:
      | disp('CONTROL ZONE DUMMY');
      | port_label('input',1,'IN');
      | port_label('input',2,'INFO');
      | port_label('output',1,'OUT');
      | port_label('output',2,'INFO');
  Out1 : Outport
  Out2 : Outport  Port=2
  wires:
  In2/1 -> MATLAB Discrete-Event System/2
  MATLAB Discrete-Event System/1 -> Out1/1
  MATLAB Discrete-Event System/2 -> Out2/1
  In1/1 -> MATLAB Discrete-Event System/1

== system Mcity/Subsystem/Subsystem1/Subsystem6 ==
  note: Right-click the system block and select "Block Parameters (MATLAB Discrete Event Systems)"
      | Choose one of the coordinators from
      | unsig_int_1_Coordinator
      | unsig_int_1_Coordinator_Dummy (choose this when testing other scenarios)
      | Double-click the system block and make sure the simulation is using "Interprated Execution" instead of "Code Generation"
  In1 : Inport
  " " : MATLABDiscreteEventSystem  InputPortMessageModes=m  OutputPortMessageModes=m  System=unsig_int_1_Coordinator_Dummy  capacity=100  SimulateUsing=Interpreted execution
      mask Type: unsig_int_1_Coordinator_Dummy
      mask Display:
      | disp('COORDINATOR DUMMY');
      | port_label('input',1,'IN');
      | port_label('output',1,'OUT');
  Out1 : Outport
  wires:
  " "/1 -> Out1/1
  In1/1 -> " "/1

== system Mcity/Subsystem/Subsystem1/Subsystem7 ==
  In1 : Inport
  MATLAB Discrete-Event System : MATLABDiscreteEventSystem  InputPortMessageModes=m  OutputPortMessageModes=m  System=unsig_int_12_RoadSegment_Dummy  capacity=400  SimulateUsing=Interpreted execution
      mask Type: unsig_int_12_RoadSegment_Dummy
      mask Display:
      | disp('LEAVE THE INTERSECTION DUMMY');
      | port_label('input',1,'IN');
      | port_label('output',1,'OUT');
  Out1 : Outport
  wires:
  MATLAB Discrete-Event System/1 -> Out1/1
  In1/1 -> MATLAB Discrete-Event System/1

== system Mcity/Subsystem/Subsystem1/Subsystem8 ==
  In1 : Inport
  MATLAB Discrete-Event System : MATLABDiscreteEventSystem  InputPortMessageModes=m  OutputPortMessageModes=m  System=unsig_int_12_RoadSegment_Dummy  capacity=400  SimulateUsing=Interpreted execution
      mask Type: unsig_int_12_RoadSegment_Dummy
      mask Display:
      | disp('LEAVE THE INTERSECTION DUMMY');
      | port_label('input',1,'IN');
      | port_label('output',1,'OUT');
  Out1 : Outport
  wires:
  MATLAB Discrete-Event System/1 -> Out1/1
  In1/1 -> MATLAB Discrete-Event System/1

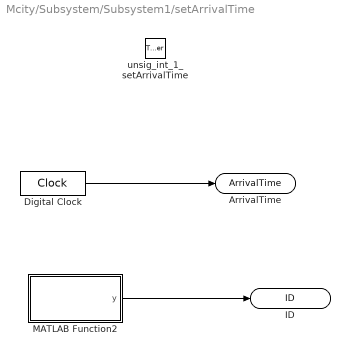
== system Mcity/Subsystem/Subsystem1/setArrivalTime ==
  unsig_int_1_setArrivalTime : TriggerPort  TriggerType=function-call  IsSimulinkFunction=on  FunctionName=unsig_int_1_setArrivalTime  FunctionVisibility=scoped  VariantControl=Variant
  Digital Clock : DigitalClock  SampleTime=-1
  MATLAB Function2 : MATLAB Function  TreatAsAtomicUnit=on
  ArrivalTime : ArgOut  DisableCoverage=on  ArgumentName=ArrivalTime
  ID : ArgOut  DisableCoverage=on  Port=2  ArgumentName=ID
  wires:
  Digital Clock/1 -> ArrivalTime/1
  MATLAB Function2/1(y) -> ID/1

== system Mcity/Subsystem/Subsystem2/Subsystem5 ==
  note: Right-click the system block and select "Block Parameters (MATLAB Discrete Event Systems)"
      | Choose one of the controllers from
      | onramp_Controller_OC (optimal control)
      | onramp_Controller_CBF (control barrier functions)
      | onramp_Controller_Dummy (choose this when testing other scenarios)
      | Double-click the system block and make sure the simulation is using "Interprated Execution" instead of "Code Generation"
  In1 : Inport
  In2 : Inport  Port=2
  MATLAB Discrete-Event System1 : MATLABDiscreteEventSystem  Description=Coordinator  InputPortMessageModes=m,m  OutputPortMessageModes=m,m  System=onramp_Controller_OC  capacity=100  simulation_step=0.01  S=30  L=400  delta=10  profiles=repmat( struct( 'control', @(t) 1, 'speed', @(t) 1, 'position', @(t) 1 ), 1001, 1 )  SimulateUsing=Interpreted execution
      mask Type: onramp_Controller_OC
      mask Display:
      | disp('FREEWAY ON-RAMP');
      | port_label('input',1,'IN');
      | port_label('input',2,'INFO');
      | port_label('output',1,'OUT');
      | port_label('output',2,'INFO');
  Out1 : Outport
  Out2 : Outport  Port=2
  wires:
  MATLAB Discrete-Event System1/2 -> Out2/1
  In2/1 -> MATLAB Discrete-Event System1/2
  In1/1 -> MATLAB Discrete-Event System1/1
  MATLAB Discrete-Event System1/1 -> Out1/1

== system Mcity/Subsystem/Subsystem2/Subsystem6 ==
  note: Right-click the system block and select "Block Parameters (MATLAB Discrete Event Systems)"
      | Choose one of the coordinators from
      | onramp_Coordinator
      | onramp_Coordinator_Dummy (choose this when testing other scenarios)
      | Double-click the system block and make sure the simulation is using "Interprated Execution" instead of "Code Generation"
  In1 : Inport
  " " : MATLABDiscreteEventSystem  InputPortMessageModes=m  OutputPortMessageModes=m  System=onramp_Coordinator  capacity=100  SimulateUsing=Interpreted execution
      mask Type: onramp_Coordinator
      mask Display:
      | disp('COORDINATOR');
      | port_label('input',1,'IN');
      | port_label('output',1,'OUT');
  Out1 : Outport
  wires:
  " "/1 -> Out1/1
  In1/1 -> " "/1

== system Mcity/Subsystem/Subsystem2/setArrivalTime ==
  onramp_setArrivalTime : TriggerPort  TriggerType=function-call  IsSimulinkFunction=on  FunctionName=onramp_setArrivalTime  FunctionVisibility=scoped  VariantControl=Variant
  Digital Clock : DigitalClock  SampleTime=-1
  MATLAB Function1 : MATLAB Function  TreatAsAtomicUnit=on
  ArrivalTime : ArgOut  DisableCoverage=on  ArgumentName=ArrivalTime
  ID : ArgOut  DisableCoverage=on  Port=2  ArgumentName=ID
  wires:
  MATLAB Function1/1(y) -> ID/1
  Digital Clock/1 -> ArrivalTime/1

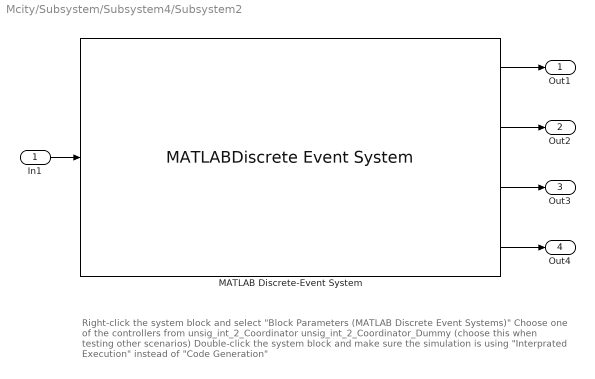
== system Mcity/Subsystem/Subsystem4/Subsystem2 ==
  note: Right-click the system block and select "Block Parameters (MATLAB Discrete Event Systems)"
      | Choose one of the controllers from
      | unsig_int_2_Coordinator
      | unsig_int_2_Coordinator_Dummy (choose this when testing other scenarios)
      | Double-click the system block and make sure the simulation is using "Interprated Execution" instead of "Code Generation"
  In1 : Inport
  MATLAB Discrete-Event System : MATLABDiscreteEventSystem  InputPortMessageModes=m  OutputPortMessageModes=m,m,m,m  System=unsig_int_2_MergingZoneCruiser_Dummy  capacity=200  SimulateUsing=Interpreted execution
      mask Type: unsig_int_2_MergingZoneCruiser_Dummy
      mask Display:
      | disp('MERGING ZONE DUMMY');
      | port_label('input',1,'CAV');
      | port_label('output',1,'TO WEST');
      | port_label('output',2,'TO SOUTH');
      | port_label('output',3,'TO EAST');
      | port_label('output',4,'TO NORTH');
  Out1 : Outport
  Out2 : Outport  Port=2
  Out3 : Outport  Port=3
  Out4 : Outport  Port=4
  wires:
  MATLAB Discrete-Event System/4 -> Out4/1
  In1/1 -> MATLAB Discrete-Event System/1
  MATLAB Discrete-Event System/3 -> Out3/1
  MATLAB Discrete-Event System/1 -> Out1/1
  MATLAB Discrete-Event System/2 -> Out2/1

== system Mcity/Subsystem/Subsystem4/Subsystem5 ==
  note: Right-click the system block and select "Block Parameters (MATLAB Discrete Event Systems)"
      | Choose one of the controllers from
      | unsig_int_2_Controller_OC (optimal control)
      | unsig_int_2_Controller_Dummy (choose this when testing other scenarios)
      | Double-click the system block and make sure the simulation is using "Interprated Execution" instead of "Code Generation"
  In1 : Inport
  In2 : Inport  Port=2
  MATLAB Discrete-Event System : MATLABDiscreteEventSystem  InputPortMessageModes=m,m  OutputPortMessageModes=m,m  System=unsig_int_2_Controller_Dummy  capacity=400  SimulateUsing=Interpreted execution
      mask Type: unsig_int_2_Controller_Dummy
      mask Display:
      | disp('CONTROL ZONE DUMMY');
      | port_label('input',1,'IN');
      | port_label('input',2,'INFO');
      | port_label('output',1,'OUT');
      | port_label('output',2,'INFO');
  Out1 : Outport
  Out2 : Outport  Port=2
  wires:
  MATLAB Discrete-Event System/1 -> Out1/1
  MATLAB Discrete-Event System/2 -> Out2/1
  In1/1 -> MATLAB Discrete-Event System/1
  In2/1 -> MATLAB Discrete-Event System/2

== system Mcity/Subsystem/Subsystem4/Subsystem6 ==
  note: Right-click the system block and select "Block Parameters (MATLAB Discrete Event Systems)"
      | Choose one of the coordinators from
      | unsig_int_2_Coordinator
      | unsig_int_2_Coordinator_Dummy (choose this when testing other scenarios)
      | Double-click the system block and make sure the simulation is using "Interprated Execution" instead of "Code Generation"
  In1 : Inport
  " " : MATLABDiscreteEventSystem  InputPortMessageModes=m  OutputPortMessageModes=m  System=unsig_int_2_Coordinator_Dummy  capacity=100  SimulateUsing=Interpreted execution
      mask Type: unsig_int_2_Coordinator_Dummy
      mask Display:
      | disp('COORDINATOR DUMMY');
      | port_label('input',1,'IN');
      | port_label('output',1,'OUT');
  Out1 : Outport
  wires:
  " "/1 -> Out1/1
  In1/1 -> " "/1

== system Mcity/Subsystem/Subsystem4/Subsystem7 ==
  In1 : Inport
  MATLAB Discrete-Event System : MATLABDiscreteEventSystem  InputPortMessageModes=m  OutputPortMessageModes=m  System=unsig_int_12_RoadSegment_Dummy  capacity=400  SimulateUsing=Interpreted execution
      mask Type: unsig_int_12_RoadSegment_Dummy
      mask Display:
      | disp('LEAVE THE INTERSECTION DUMMY');
      | port_label('input',1,'IN');
      | port_label('output',1,'OUT');
  Out1 : Outport
  wires:
  MATLAB Discrete-Event System/1 -> Out1/1
  In1/1 -> MATLAB Discrete-Event System/1

== system Mcity/Subsystem/Subsystem4/Subsystem8 ==
  In1 : Inport
  MATLAB Discrete-Event System : MATLABDiscreteEventSystem  InputPortMessageModes=m  OutputPortMessageModes=m  System=unsig_int_12_RoadSegment_Dummy  capacity=400  SimulateUsing=Interpreted execution
      mask Type: unsig_int_12_RoadSegment_Dummy
      mask Display:
      | disp('LEAVE THE INTERSECTION DUMMY');
      | port_label('input',1,'IN');
      | port_label('output',1,'OUT');
  Out1 : Outport
  wires:
  MATLAB Discrete-Event System/1 -> Out1/1
  In1/1 -> MATLAB Discrete-Event System/1

== system Mcity/Subsystem/Subsystem4/Subsystem9 ==
  In1 : Inport
  MATLAB Discrete-Event System : MATLABDiscreteEventSystem  InputPortMessageModes=m  OutputPortMessageModes=m  System=unsig_int_12_RoadSegment_Dummy  capacity=400  SimulateUsing=Interpreted execution
      mask Type: unsig_int_12_RoadSegment_Dummy
      mask Display:
      | disp('LEAVE THE INTERSECTION DUMMY');
      | port_label('input',1,'IN');
      | port_label('output',1,'OUT');
  Out1 : Outport
  wires:
  MATLAB Discrete-Event System/1 -> Out1/1
  In1/1 -> MATLAB Discrete-Event System/1

== system Mcity/Subsystem/Subsystem4/setArrivalTime ==
  unsig_int_2_setArrivalTime : TriggerPort  TriggerType=function-call  IsSimulinkFunction=on  FunctionName=unsig_int_2_setArrivalTime  FunctionVisibility=scoped  VariantControl=Variant
  Digital Clock : DigitalClock  SampleTime=-1
  MATLAB Function : MATLAB Function  TreatAsAtomicUnit=on
  ArrivalTime : ArgOut  DisableCoverage=on  ArgumentName=ArrivalTime
  ID : ArgOut  DisableCoverage=on  Port=2  ArgumentName=ID
  wires:
  Digital Clock/1 -> ArrivalTime/1
  MATLAB Function/1(y) -> ID/1

== matlab function Mcity/Subsystem/Subsystem/setArrivalTime/MATLAB Function1 ==
  data: y output; sig_int_FF data_store_memory
function y = getID()
global sig_int_FF

sig_int_FF = sig_int_FF + 1;
y = sig_int_FF;

== matlab function Mcity/Subsystem/Subsystem2/setArrivalTime/MATLAB Function1 ==
  data: y output; onramp_FF data_store_memory
function y = getID()
global onramp_FF

onramp_FF = onramp_FF + 1;
y = onramp_FF;

== matlab function Mcity/Subsystem/Subsystem1/setArrivalTime/MATLAB Function2 ==
  data: y output; unsig_int_1_FF data_store_memory
function y = getID
global unsig_int_1_FF

unsig_int_1_FF = unsig_int_1_FF + 1;
y = unsig_int_1_FF;

== matlab function Mcity/Subsystem/Subsystem4/setArrivalTime/MATLAB Function ==
  data: y output; unsig_int_2_FF data_store_memory
function y = getID
global unsig_int_2_FF

unsig_int_2_FF = unsig_int_2_FF + 1;
y = unsig_int_2_FF;
